simulink model "sim_3dof_model"  (R2015b)
settings: Solver=VariableStepAuto  StartTime=0.0  StopTime=10  RelTol=1e-3
libraries: cstblocks x4
settings Model: Creator=lbromo12  LastModifiedBy=alvaro

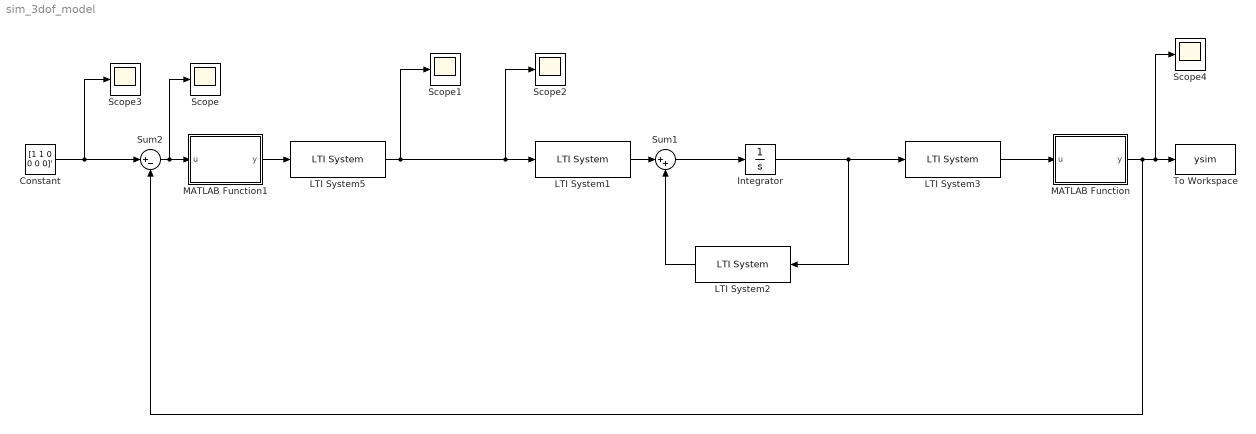
== system sim_3dof_model ==
  Constant : Constant  Value=[1 1 0 0 0 0]'
  Integrator : Integrator
  LTI System1 : cstblocks/LTI System  sys=B  IC=[]
  LTI System2 : cstblocks/LTI System  sys=A  IC=[]
  LTI System3 : cstblocks/LTI System  sys=C  IC=[]
  LTI System5 : cstblocks/LTI System  sys=LQR  IC=[]
  MATLAB Function : MATLAB Function  TreatAsAtomicUnit=on
  MATLAB Function1 : MATLAB Function  TreatAsAtomicUnit=on
  Scope{,1..4} (5 alike) : Scope
  Sum1 : Sum  Inputs=|++
  Sum2 : Sum  Inputs=|+-
  To Workspace : ToWorkspace  VariableName=ysim  SaveFormat=Timeseries  SampleTime=-1
  wires:
  LTI System5/1 -> Scope2/1, LTI System1/1, Scope1/1
  LTI System2/1 -> Sum1/2
  LTI System1/1 -> Sum1/1
  Sum2/1 -> Scope/1, MATLAB Function1/1(u)
  Constant/1 -> Scope3/1, Sum2/1
  MATLAB Function1/1(y) -> LTI System5/1
  LTI System3/1 -> MATLAB Function/1(u)
  Sum1/1 -> Integrator/1
  MATLAB Function/1(y) -> Sum2/2, Scope4/1, To Workspace/1
  Integrator/1 -> LTI System3/1, LTI System2/1

== matlab function sim_3dof_model/MATLAB Function1 ==
  data: u input; y output
function y   = NED2BODY(u)
    psi = u(3);
    P = [
        cos(psi) -sin(psi) 0 0 0 0;
        sin(psi) cos(psi) 0 0 0 0;
        0 0 1 0 0 0;
        zeros(3) eye(3);
        ];
    
    y = P'*u;

== matlab function sim_3dof_model/MATLAB Function ==
  data: u input; y output
function y  = BODY2NED(u)
    psi = u(3);
    P = [
        cos(psi) -sin(psi) 0 0 0 0;
        sin(psi) cos(psi) 0 0 0 0;
        0 0 1 0 0 0;
        zeros(3) eye(3);
        ]
    
    y = P*u;
